simulink model "Lab1_parameter_estimation_student_Multi"  (R2024b)
settings: Solver=FixedStepAuto  StartTime=0  StopTime=60  FixedStep=0.0001  RelTol=1e-3
values from neighbouring files (symbols this model uses):
  motor_B = 0.0001    [Lab1_motor_params_student.m]    (also in Lab1_motor_params_student_multi.m)
  motor_Eff = 0.5    [Lab1_motor_params_student.m]    (also in Lab1_motor_params_student_multi.m)
  motor_J = 0.001    [Lab1_motor_params_student.m]    (also in Lab1_motor_params_student_multi.m)
  motor_Ke = 0.05    [Lab1_motor_params_student.m]    (also in Lab1_motor_params_student_multi.m)
  motor_L = 0.0254006445    [Lab1_motor_params_student.m]    (also in Lab1_motor_params_student_multi.m = 0.0291360334)
  motor_R = 0.98275    [Lab1_motor_params_student.m]    (also in Lab1_motor_params_student_multi.m = 1.12727)
libraries: simulink x1
settings Model: Creator=tanawatp  LastModifiedBy=acer
settings RTWCC: GPUComputeCapability=3.5

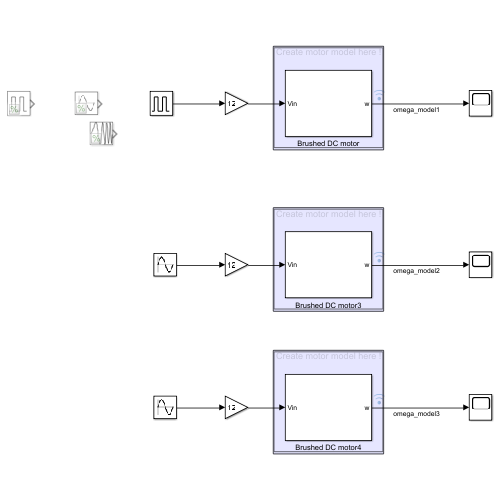
[thumbnail: Simulink's stored preview of the top-level diagram]
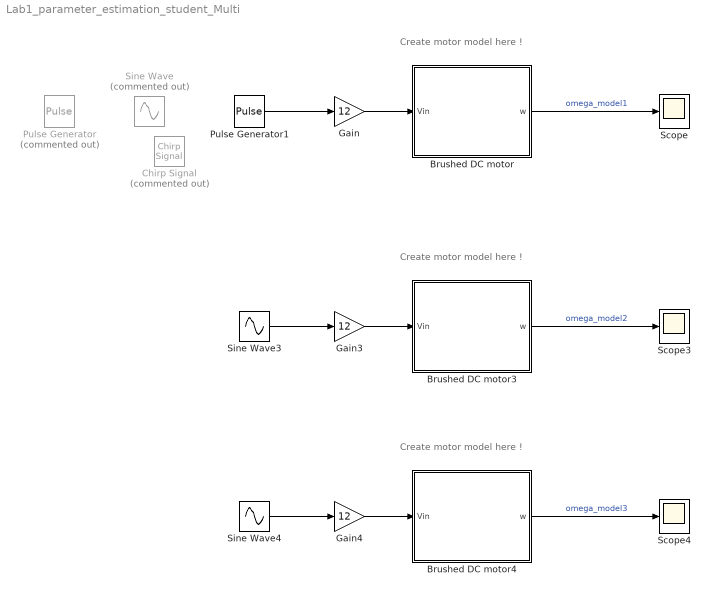
== system Lab1_parameter_estimation_student_Multi ==
  note: Create motor model here !
  note: Create motor model here !
  note: Create motor model here !
  Brushed DC motor : Subsystem
  Brushed DC motor3 : Subsystem
  Brushed DC motor4 : Subsystem
  Chirp Signal : simulink/Sources/Chirp Signal  Commented=on  f1=0  T=60  f2=0.5
  Gain : Gain  Gain=12
  Gain3 : Gain  Gain=12
  Gain4 : Gain  Gain=12
  Pulse Generator : DiscretePulseGenerator  Commented=on  PulseType=Time based  PulseWidth=50
  Pulse Generator1 : DiscretePulseGenerator  PulseType=Time based  PulseWidth=50
  Scope : Scope
  Scope3 : Scope
  Scope4 : Scope
  Sine Wave : Sin  Commented=on  SampleTime=0
  Sine Wave3 : Sin  SampleTime=0
  Sine Wave4 : Sin  Frequency=4  SampleTime=0
  wires:
  Brushed DC motor/1(w) -> Scope/1  "omega_model1"
  Pulse Generator1/1 -> Gain/1
  Gain/1 -> Brushed DC motor/1(Vin)
  Gain3/1 -> Brushed DC motor3/1(Vin)
  Sine Wave3/1 -> Gain3/1
  Brushed DC motor3/1(w) -> Scope3/1  "omega_model2"
  Brushed DC motor4/1(w) -> Scope4/1  "omega_model3"
  Sine Wave4/1 -> Gain4/1
  Gain4/1 -> Brushed DC motor4/1(Vin)

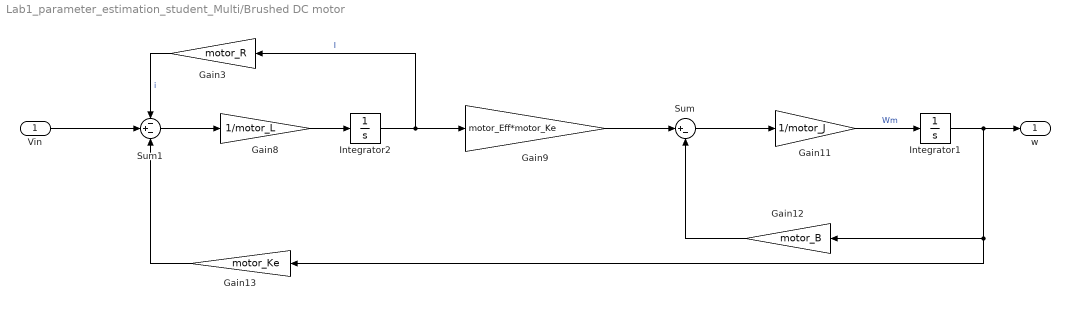
== system Lab1_parameter_estimation_student_Multi/Brushed DC motor ==
  Vin : Inport
  Gain11 : Gain  Gain=1/motor_J
  Gain12 : Gain  Gain=motor_B
  Gain13 : Gain  Gain=motor_Ke
  Gain3 : Gain  Gain=motor_R
  Gain8 : Gain  Gain=1/motor_L
  Gain9 : Gain  Gain=motor_Eff*motor_Ke
  Integrator1 : Integrator
  Integrator2 : Integrator
  Sum : Sum  Inputs=|+-
  Sum1 : Sum  Inputs=-+-
  w : Outport
  wires:
  Gain9/1 -> Sum/1
  Sum/1 -> Gain11/1
  Gain12/1 -> Sum/2
  Gain11/1 -> Integrator1/1  "Wm"
  Integrator1/1 -> Gain12/1, Gain13/1, w/1
  Vin/1 -> Sum1/2
  Gain3/1 -> Sum1/1  "i"
  Gain13/1 -> Sum1/3
  Sum1/1 -> Gain8/1
  Gain8/1 -> Integrator2/1
  Integrator2/1 -> Gain3/1, Gain9/1  "I"

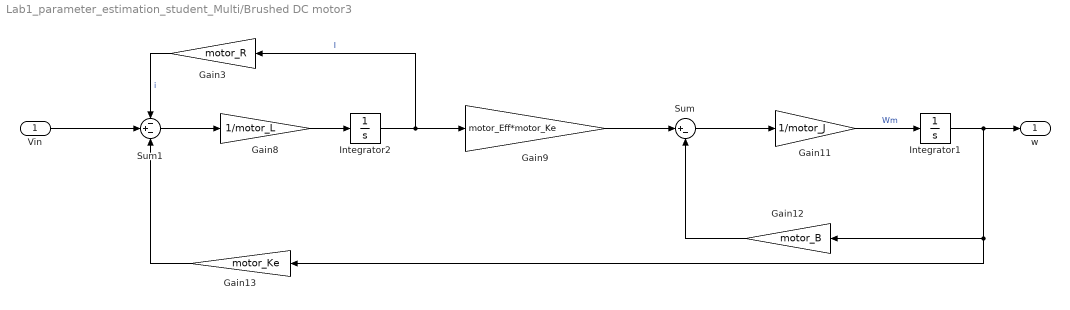
== system Lab1_parameter_estimation_student_Multi/Brushed DC motor3 ==
  Vin : Inport
  Gain11 : Gain  Gain=1/motor_J
  Gain12 : Gain  Gain=motor_B
  Gain13 : Gain  Gain=motor_Ke
  Gain3 : Gain  Gain=motor_R
  Gain8 : Gain  Gain=1/motor_L
  Gain9 : Gain  Gain=motor_Eff*motor_Ke
  Integrator1 : Integrator
  Integrator2 : Integrator
  Sum : Sum  Inputs=|+-
  Sum1 : Sum  Inputs=-+-
  w : Outport
  wires:
  Integrator2/1 -> Gain9/1, Gain3/1  "I"
  Gain8/1 -> Integrator2/1
  Sum1/1 -> Gain8/1
  Gain13/1 -> Sum1/3
  Gain3/1 -> Sum1/1  "i"
  Vin/1 -> Sum1/2
  Integrator1/1 -> w/1, Gain13/1, Gain12/1
  Gain11/1 -> Integrator1/1  "Wm"
  Gain12/1 -> Sum/2
  Sum/1 -> Gain11/1
  Gain9/1 -> Sum/1

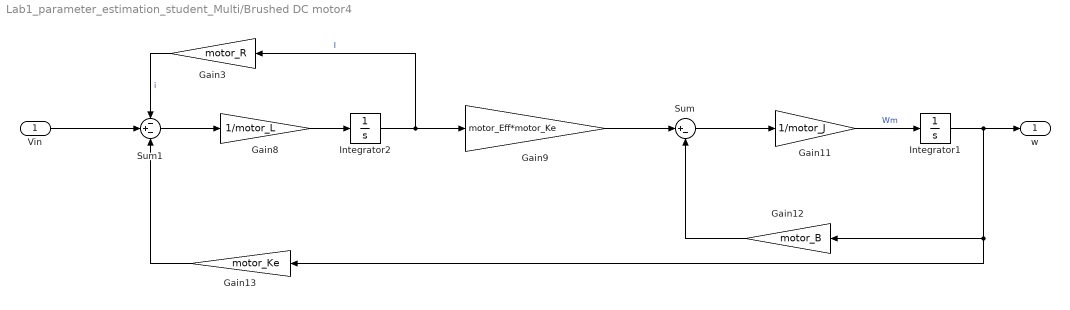
== system Lab1_parameter_estimation_student_Multi/Brushed DC motor4 ==
  Vin : Inport
  Gain11 : Gain  Gain=1/motor_J
  Gain12 : Gain  Gain=motor_B
  Gain13 : Gain  Gain=motor_Ke
  Gain3 : Gain  Gain=motor_R
  Gain8 : Gain  Gain=1/motor_L
  Gain9 : Gain  Gain=motor_Eff*motor_Ke
  Integrator1 : Integrator
  Integrator2 : Integrator
  Sum : Sum  Inputs=|+-
  Sum1 : Sum  Inputs=-+-
  w : Outport
  wires:
  Gain9/1 -> Sum/1
  Sum/1 -> Gain11/1
  Gain12/1 -> Sum/2
  Gain11/1 -> Integrator1/1  "Wm"
  Integrator1/1 -> Gain12/1, Gain13/1, w/1
  Vin/1 -> Sum1/2
  Gain3/1 -> Sum1/1  "i"
  Gain13/1 -> Sum1/3
  Sum1/1 -> Gain8/1
  Gain8/1 -> Integrator2/1
  Integrator2/1 -> Gain3/1, Gain9/1  "I"
